simulink model "TaskSolution"  (R2018b)
settings: Solver=ode45  StartTime=0.0  StopTime=20  MaxStep=1e-3  RelTol=1e-3
values from neighbouring files (symbols this model uses):
  b1 = 2 * zeta * sqrt(K * m1)    [SimulateModel.m]
  b2 = 2 * zeta * sqrt(K * m2)    [SimulateModel.m]
  K = 350    [SimulateModel.m]
  Kd = 30    [SimulateModel.m]
  Kp = 200    [SimulateModel.m]
  m1 = 0.6    [SimulateModel.m]
  m2 = 1.0    (= 1)    [SimulateModel.m]
  x1_0 = 5    [SimulateModel.m]
  x1Dot_0 = 0    [SimulateModel.m]
  x2_0 = 0    [SimulateModel.m]
  x2Dot_0 = 0    [SimulateModel.m]
  x_ref = 7    [SimulateModel.m]
settings Model: Creator=madho  LastModifiedBy=madho
settings DataIOCC: ReturnWorkspaceOutputs=on
settings DebuggingCC: UnconnectedInputMsg=none  UnconnectedOutputMsg=none  UnconnectedLineMsg=none
settings ModelReferenceCC: EnableRefExpFcnMdlSchedulingChecks=off
settings RTWCC: Description=Generic Real-Time Target

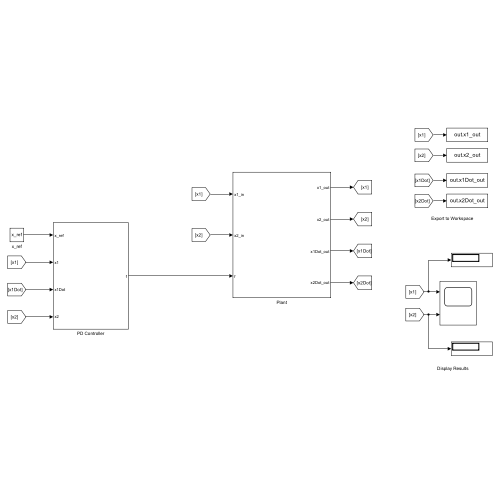
[thumbnail: Simulink's stored preview of the top-level diagram]
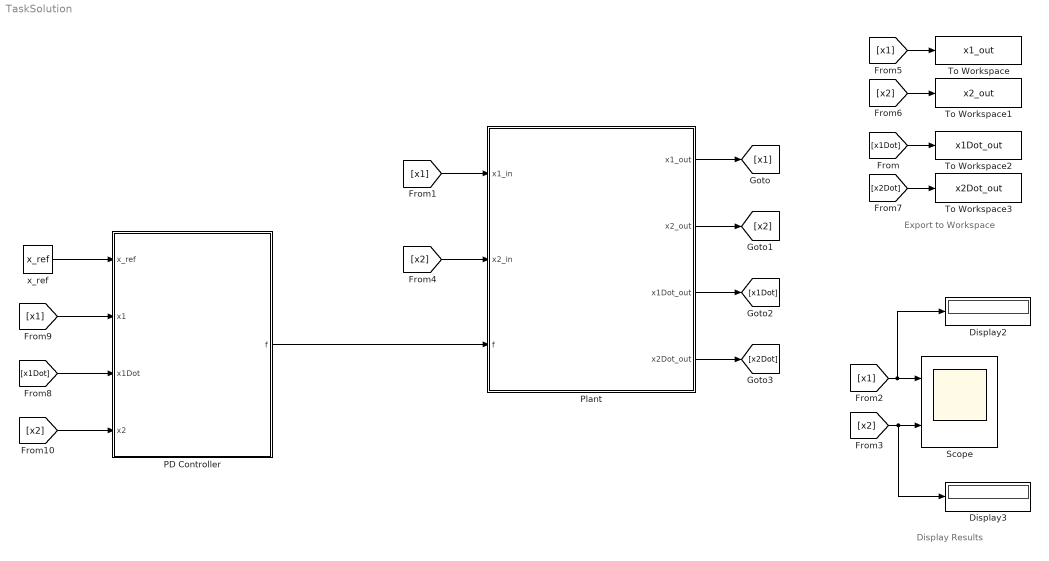
== system TaskSolution ==
  note: Export to Workspace
  note: Display Results
  Display2 : Display
  Display3 : Display
  PD Controller : Subsystem
  Plant : Subsystem
  Scope : Scope  NumInputPorts=2
  To Workspace : ToWorkspace  VariableName=x1_out  SampleTime=-1
  To Workspace1 : ToWorkspace  VariableName=x2_out  SampleTime=-1
  To Workspace2 : ToWorkspace  VariableName=x1Dot_out  SampleTime=-1
  To Workspace3 : ToWorkspace  VariableName=x2Dot_out  SampleTime=-1
  x_ref : Constant  Value=x_ref
  wires:
  [x1] -> Display2/1, Scope/1
  [x2] -> Display3/1, Scope/2
  [x1] -> Plant/1(x1_in)
  [x2] -> Plant/2(x2_in)
  Plant/2(x2_out) -> [x2]
  Plant/1(x1_out) -> [x1]
  [x1] -> To Workspace/1
  [x2] -> To Workspace1/1
  [x2Dot] -> To Workspace3/1
  [x1Dot] -> To Workspace2/1
  Plant/4(x2Dot_out) -> [x2Dot]
  Plant/3(x1Dot_out) -> [x1Dot]
  PD Controller/1(f) -> Plant/3(f)
  [x1Dot] -> PD Controller/3(x1Dot)
  [x1] -> PD Controller/2(x1)
  x_ref/1 -> PD Controller/1(x_ref)
  [x2] -> PD Controller/4(x2)

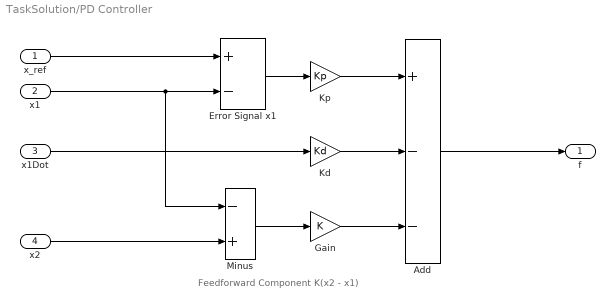
== system TaskSolution/PD Controller ==
  note: Feedforward Component K(x2 - x1)
  x_ref : Inport
  x1 : Inport  Port=2
  x1Dot : Inport  Port=3
  x2 : Inport  Port=4
  Add : Sum  Inputs=+--
  Error Signal x1 : Sum  Inputs=+-
  Gain : Gain  Gain=K
  Kd : Gain  Gain=Kd
  Kp : Gain  Gain=Kp
  Minus : Sum  Inputs=-+
  f : Outport
  wires:
  Add/1 -> f/1
  Error Signal x1/1 -> Kp/1
  x1Dot/1 -> Kd/1
  Kd/1 -> Add/2
  x_ref/1 -> Error Signal x1/1
  x1/1 -> Minus/1, Error Signal x1/2
  Kp/1 -> Add/1
  Gain/1 -> Add/3
  Minus/1 -> Gain/1
  x2/1 -> Minus/2

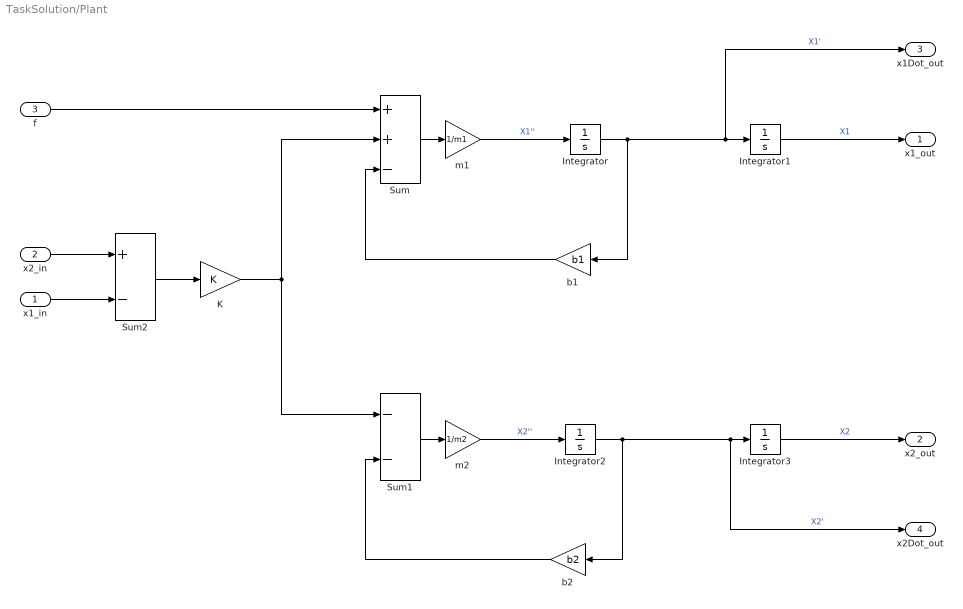
== system TaskSolution/Plant ==
  x1_in : Inport
  x2_in : Inport  Port=2
  f : Inport  Port=3
  Integrator : Integrator  InitialCondition=x1Dot_0
  Integrator1 : Integrator  InitialCondition=x1_0
  Integrator2 : Integrator  InitialCondition=x2Dot_0
  Integrator3 : Integrator  InitialCondition=x2_0
  K : Gain  Gain=K
  Sum : Sum  Inputs=++-
  Sum1 : Sum  Inputs=--
  Sum2 : Sum  Inputs=+-
  b1 : Gain  Gain=b1
  b2 : Gain  Gain=b2
  m1 : Gain  Gain=1/m1
  m2 : Gain  Gain=1/m2
  x1_out : Outport
  x2_out : Outport  Port=2
  x1Dot_out : Outport  Port=3
  x2Dot_out : Outport  Port=4
  wires:
  Integrator2/1 -> b2/1, x2Dot_out/1, Integrator3/1  "X2'"
  Sum/1 -> m1/1
  m2/1 -> Integrator2/1  "X2''"
  Integrator/1 -> b1/1, x1Dot_out/1, Integrator1/1  "X1'"
  Integrator1/1 -> x1_out/1  "X1"
  Integrator3/1 -> x2_out/1  "X2"
  K/1 -> Sum/2, Sum1/1
  Sum2/1 -> K/1
  b2/1 -> Sum1/2
  m1/1 -> Integrator/1  "X1''"
  Sum1/1 -> m2/1
  x2_in/1 -> Sum2/1
  x1_in/1 -> Sum2/2
  b1/1 -> Sum/3
  f/1 -> Sum/1
